simulink library "RollRefAssessLib"  (R2016a)
settings: Solver=VariableStepAuto  StartTime=0.0  StopTime=10.0  RelTol=1e-3
libraries: simulink x8, sldvlib x4
settings Model: Creator=The MathWorks, Inc.  LastModifiedBy=The MathWorks, Inc.
settings DataIOCC: LimitDataPoints=on
settings DebuggingCC: AllowSymbolicDim=off
settings HardwareCC: ProdWordSize=32
settings ModelReferenceCC: PropagateSignalLabelsOutOfModel=off
settings GRTTargetCC: GeneratePreprocessorConditionals=Use local settings

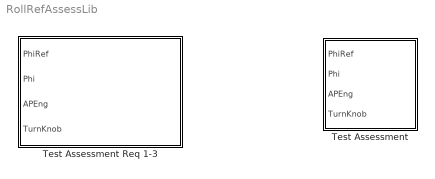
== system RollRefAssessLib ==
  Test Assessment : State Transition Table  TreatAsAtomicUnit=on
  Test Assessment Req 1-3 : Subsystem

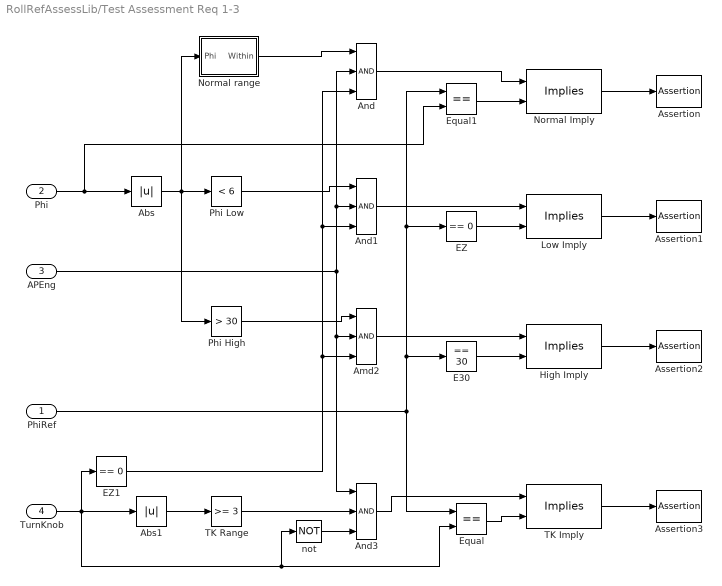
== system RollRefAssessLib/Test Assessment Req 1-3 ==
  PhiRef : Inport
  Phi : Inport  Port=2
  APEng : Inport  Port=3
  TurnKnob : Inport  Port=4
  Abs : Abs
  Abs1 : Abs
  Amd2 : Logic  Inputs=3  AllPortsSameDT=off  OutDataTypeStr=boolean
  And : Logic  Inputs=3  AllPortsSameDT=off  OutDataTypeStr=boolean
  And1 : Logic  Inputs=3  AllPortsSameDT=off  OutDataTypeStr=boolean
  And3 : Logic  Inputs=3  AllPortsSameDT=off  OutDataTypeStr=boolean
  Assertion : Assertion  AssertionFailFcn=disp(sprintf('\nPhiRef must = Phi when Phi in normal range.'))  StopWhenAssertionFail=off
  Assertion1 : Assertion  AssertionFailFcn=disp(sprintf('\nPhiRef must = 0 when Phi < 6 deg.'))  StopWhenAssertionFail=off
  Assertion2 : Assertion  AssertionFailFcn=disp(sprintf('\nFailure of high limit test.\nPhiRef must = 0 when Phi > 30 deg.'))  StopWhenAssertionFail=off
  Assertion3 : Assertion  AssertionFailFcn=disp(sprintf('\nPhiRef must = TK value when TK > 3 deg.'))  StopWhenAssertionFail=off
  E30 : simulink/Logic and Bit Operations/Compare To Constant  relop===  const=30  OutDataTypeStr=boolean
  EZ : simulink/Logic and Bit Operations/Compare To Zero  relop===  OutDataTypeStr=boolean
  EZ1 : simulink/Logic and Bit Operations/Compare To Zero  relop===  OutDataTypeStr=boolean
  Equal : RelationalOperator  Operator===  OutDataTypeStr=boolean
  Equal1 : RelationalOperator  Operator===  OutDataTypeStr=boolean
  High Imply : sldvlib/Verification Utilities/Implies
  Low Imply : sldvlib/Verification Utilities/Implies
  Normal Imply : sldvlib/Verification Utilities/Implies
  Normal range : Subsystem
  Phi High : simulink/Logic and Bit Operations/Compare To Constant  relop=>  const=30  OutDataTypeStr=boolean
  Phi Low : simulink/Logic and Bit Operations/Compare To Constant  relop=<  const=6  OutDataTypeStr=boolean
  TK Imply : sldvlib/Verification Utilities/Implies
  TK Range : simulink/Logic and Bit Operations/Compare To Constant  relop=>=  const=3  OutDataTypeStr=boolean
  not : Logic  Operator=NOT  Inputs=1  AllPortsSameDT=off  OutDataTypeStr=boolean
  wires:
  APEng/1 -> And3/1, Amd2/2, And/2, And1/2
  Phi/1 -> Equal1/2, Abs/1
  Phi Low/1 -> And1/1
  EZ/1 -> Low Imply/2
  PhiRef/1 -> E30/1, Equal1/1, EZ/1, Equal/1
  And1/1 -> Low Imply/1
  Phi High/1 -> Amd2/1
  E30/1 -> High Imply/2
  Amd2/1 -> High Imply/1
  Abs/1 -> Normal range/1(Phi), Phi High/1, Phi Low/1
  Abs1/1 -> TK Range/1
  TK Range/1 -> And3/2
  And3/1 -> TK Imply/1
  Equal/1 -> TK Imply/2
  Normal range/1(Within) -> And/1
  Equal1/1 -> Normal Imply/2
  And/1 -> Normal Imply/1
  Low Imply/1 -> Assertion1/1
  High Imply/1 -> Assertion2/1
  TK Imply/1 -> Assertion3/1
  Normal Imply/1 -> Assertion/1
  EZ1/1 -> Amd2/3, And1/3, And/3
  TurnKnob/1 -> EZ1/1, not/1, Equal/2, Abs1/1
  not/1 -> And3/3

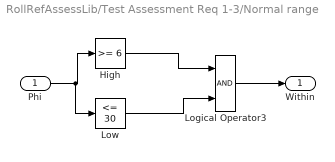
== system RollRefAssessLib/Test Assessment Req 1-3/Normal range ==
  Phi : Inport
  High : simulink/Logic and Bit Operations/Compare To Constant  relop=>=  const=6  OutDataTypeStr=boolean
  Logical Operator3 : Logic  AllPortsSameDT=off  OutDataTypeStr=boolean
  Low : simulink/Logic and Bit Operations/Compare To Constant  relop=<=  const=30  OutDataTypeStr=boolean
  Within : Outport
  wires:
  Low/1 -> Logical Operator3/2
  Phi/1 -> Low/1, High/1
  High/1 -> Logical Operator3/1
  Logical Operator3/1 -> Within/1

== stateflow chart RollRefAssessLib/Test Assessment ==
  settings: stateMachineType=SIMPLIFIED_MACHINE
  state GlobalAssessment
    state NormalRange
      verify(PhiRef == Phi,'Simulink:verify_normal','PhiRef must equal Phi for normal operation')
    state BelowLowLimit
      verify(PhiRef == 0,'Simulink:verify_low','PhiRef must equal 0 for low angle operation')
    state ExceedPosLimit
      verify(PhiRef == 30,'Simulink:verify_high','PhiRef must equal 30 for high pos angle operation')
    state ExceedNegLimit
      verify(PhiRef == -30,'Simulink:verify_high','PhiRef must equal -30 for high neg angle operation')
    state TurnKnobAssessments
      state BelowLowTKLimit
        verify(PhiRef == 0,'Simulink:verifyTKLow','PhiRef must equal 0 for low TK operation')
      state NormalTKLimit
        verify(PhiRef == TurnKnob,'Simulink:verifyTKNormal','PhiRef must equal TurnKnob for normal TK operation')
      state Else2
      (default) -> (junction 102)
      TurnKnobAssessments -> (junction 102)
      (junction 102) -> (junction 103) [order 1] : [abs(Phi) < 3]
      (junction 103) -> BelowLowTKLimit [order 1] : [~in(BelowLowTKLimit)]
      (junction 102) -> (junction 113) [order 2]
      (junction 103) -> (junction 106) [order 2]
      (junction 113) -> (junction 114) [order 1] : [abs(Phi) >=3 && Phi <= 30]
      (junction 114) -> NormalTKLimit [order 1] : [~in(NormalTKLimit)]
      (junction 114) -> (junction 117) [order 2]
      (junction 120) -> (junction 121)
      (junction 121) -> Else2 [order 1] : [~in(Else2)]
      (junction 121) -> (junction 124) [order 2]
      (junction 113) -> (junction 120) [order 2]
    state Else1
    GlobalAssessment -> (junction 22)
    (default) -> (junction 22)
    (junction 22) -> (junction 23) [order 1] : [(abs(Phi) >= 6 && Phi <= 30) && APEng == true && TurnKnob == false]
    (junction 23) -> NormalRange [order 1] : [~in(NormalRange)]
    (junction 22) -> (junction 46) [order 2]
    (junction 23) -> (junction 26) [order 2]
    (junction 46) -> (junction 47) [order 1] : [abs(Phi) < 6 && APEng == true && TurnKnob == false]
    (junction 47) -> BelowLowLimit [order 1] : [~in(BelowLowLimit)]
    (junction 46) -> (junction 73) [order 2]
    (junction 47) -> (junction 50) [order 2]
    (junction 73) -> (junction 74) [order 1] : [Phi > 30 && APEng == true && TurnKnob == false]
    (junction 74) -> ExceedPosLimit [order 1] : [~in(ExceedPosLimit)]
    (junction 73) -> (junction 84) [order 2]
    (junction 74) -> (junction 77) [order 2]
    (junction 84) -> (junction 85) [order 1] : [Phi < -30 && APEng == true && TurnKnob == false]
    (junction 85) -> ExceedNegLimit [order 1] : [~in(ExceedNegLimit)]
    (junction 84) -> (junction 62) [order 2]
    (junction 85) -> (junction 88) [order 2]
    (junction 62) -> (junction 63) [order 1] : [APEng == true && TurnKnob == true]
    (junction 63) -> TurnKnobAssessments [order 1] : [~in(TurnKnobAssessments)]
    (junction 62) -> (junction 31) [order 2]
    (junction 63) -> (junction 66) [order 2]
    (junction 31) -> (junction 32)
    (junction 32) -> Else1 [order 1] : [~in(Else1)]
    (junction 32) -> (junction 35) [order 2]
  (default) -> GlobalAssessment
  data: PhiRef input; Phi input; APEng input; TurnKnob input
